simulink model "problem4"  (R2020a)
settings: Solver=ode15s  StartTime=0.0  StopTime=0.2  RelTol=1e-3
model workspace (MAT data in the model file):
  kd = 1
  ki = 1.4
  kp = 0.1
undefined symbols (not defined in the file): b, J, K, L, R
settings Model: DataDictionary=datadict.sldd  Creator=Jake  LastModifiedBy=Jake

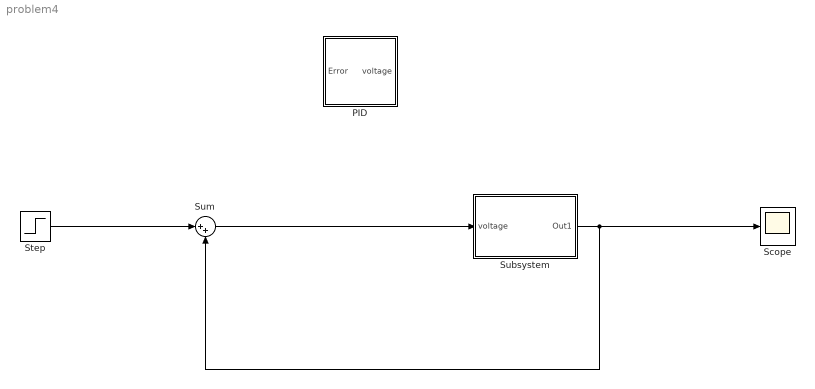
== system problem4 ==
  PID : Subsystem
  Scope : Scope
  Step : Step  Time=0  SampleTime=0
  Subsystem : Subsystem
  Sum : Sum  Inputs=|++
  wires:
  Subsystem/1(Out1) -> Sum/2, Scope/1
  Step/1 -> Sum/1
  Sum/1 -> Subsystem/1(voltage)

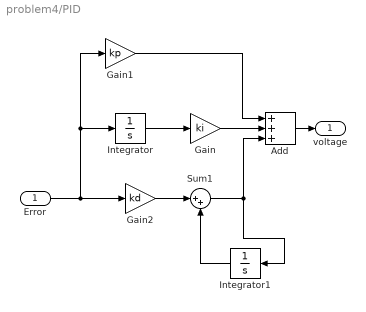
== system problem4/PID ==
  Error : Inport
  Add : Sum  Inputs=+++
  Gain : Gain  Gain=ki
  Gain1 : Gain  Gain=kp
  Gain2 : Gain  Gain=kd
  Integrator : Integrator
  Integrator1 : Integrator
  Sum1 : Sum  Inputs=|++
  voltage : Outport
  wires:
  Gain/1 -> Add/2
  Integrator/1 -> Gain/1
  Error/1 -> Gain2/1, Gain1/1, Integrator/1
  Sum1/1 -> Add/3, Integrator1/1
  Gain2/1 -> Sum1/1
  Integrator1/1 -> Sum1/2
  Gain1/1 -> Add/1
  Add/1 -> voltage/1

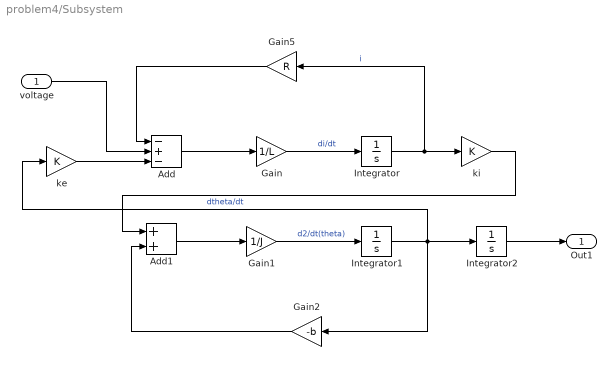
== system problem4/Subsystem ==
  voltage : Inport
  Add : Sum  Inputs=-+-
  Add1 : Sum
  Gain : Gain  Gain=1/L
  Gain1 : Gain  Gain=1/J
  Gain2 : Gain  Gain=-b
  Gain5 : Gain  Gain=R
  Integrator : Integrator
  Integrator1 : Integrator
  Integrator2 : Integrator
  ke : Gain  Gain=K
  ki : Gain  Gain=K
  Out1 : Outport
  wires:
  ke/1 -> Add/3
  Add1/1 -> Gain1/1
  Integrator1/1 -> Integrator2/1, Gain2/1, ke/1  "dtheta/dt"
  Add/1 -> Gain/1
  Integrator/1 -> Gain5/1, ki/1  "i"
  Gain/1 -> Integrator/1  "di/dt"
  Gain1/1 -> Integrator1/1  "d2/dt(theta)"
  Gain2/1 -> Add1/2
  voltage/1 -> Add/2
  ki/1 -> Add1/1
  Gain5/1 -> Add/1
  Integrator2/1 -> Out1/1
